simulink model "dyn1"  (R2021b)
settings: Solver=VariableStepAuto  StartTime=0.0  StopTime=10.0  RelTol=1e-3
InitFcn:
  | m=5;
  | I=[0.5 0 0; 0 0.5 0; 0 0 1];
  | c_t=0.02;
  | c_m=0.005;
  | h_i=10;
  | g=9.80665;
  | rho=1;
  | omega_hover=sqrt(m*g/(4*0.5*c_t));
  | dlgtitle= 'Flight Mode Selection';
  | prompt='Select the flight mode:';
  | list={'Hover', 'Underactuation by 10%', 'Overactuation of Only Rear Motor by 10%'};
  | [casee,~]=listdlg('PromptString',prompt,'ListString',list,'ListSize',[240,80],'InitialValue',1,'Name','Mode Selection','OKString','Select','SelectionMode','single');
  | if casee==1
  |     omega1=omega_hover;
  |     omega2=omega_hover;
  |     omega3=omega_hover;
  |     omega4=omega_hover;
  | elseif casee==2
  |     omega1=0.9*omega_hover;
  |     omega2=0.9*omega_hover;
  |     omega3=0.9*omega_hover;
  |     omega4=0.9*omega_hover;
  | elseif casee==3
  |     omega1=omega_hover;
  |     omega2=omega_hover;
  |     omega3=1.1*omega_hover;
  |     omega4=omega_hover;
  | end
undefined symbols (not defined in the file or in its folder): X, Y, Z
libraries: sm_lib x32, nesl_utility x11
(part 2 of 2)

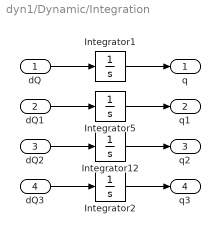
== system dyn1/Dynamic/Integration ==
  dQ : Inport
  dQ1 : Inport  Port=2
  dQ2 : Inport  Port=3
  dQ3 : Inport  Port=4
  Integrator1 : Integrator  InitialCondition=1
  Integrator12 : Integrator
  Integrator2 : Integrator
  Integrator5 : Integrator
  q : Outport
  q1 : Outport  Port=2
  q2 : Outport  Port=3
  q3 : Outport  Port=4
  wires:
  Integrator1/1 -> q/1
  Integrator5/1 -> q1/1
  dQ/1 -> Integrator1/1
  Integrator12/1 -> q2/1
  dQ1/1 -> Integrator5/1
  dQ2/1 -> Integrator12/1
  dQ3/1 -> Integrator2/1
  Integrator2/1 -> q3/1

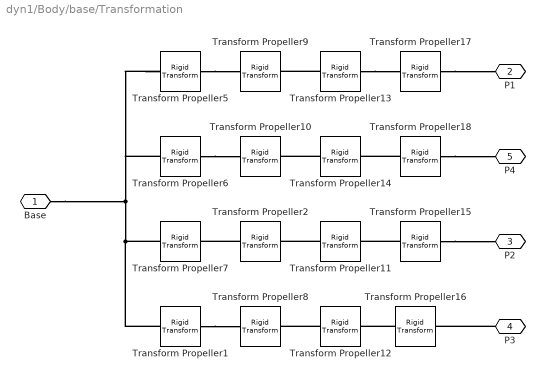
== system dyn1/Body/base/Transformation ==
  Transform Propeller1 : sm_lib/Frames and Transforms/Rigid Transform  TranslationMethod=None  TranslationStandardOffset=45  TranslationLengthUnit=mm  TranslationStandardAxis=+Z  TranslationCartesianOffset=[0 0 -20]  TranslationROffset=0  TranslationROffsetUnits=m  TranslationZOffset=0  TranslationZOffsetUnits=m  TranslationThetaOffset=0  TranslationThetaOffsetUnits=deg  RotationMethod=StandardAxis  RotationAngleUnits=deg  RotationStandardAxis=+Z  RotationAngle=-135  RotationArbitraryAxis=[0 0 1]  FollAlignAxisA=+X  BaseAlignAxisA=+Y  FollAlignAxisB=+Y  BaseAlignAxisB=+Z  RotationSequenceAxes=FollowerAxes  RotationSequence=XYX  RotationSequenceAngles=[0 0 0]  RotationSequenceAnglesUnits=deg  RotationMatrix=[1 0 0; 0 1 0; 0 0 1]
  Transform Propeller{2,8..10} (4 alike) : sm_lib/Frames and Transforms/Rigid Transform  TranslationMethod=StandardAxis  TranslationStandardOffset=60.2  TranslationLengthUnit=mm  TranslationStandardAxis=+X  TranslationCartesianOffset=[0 0 -20]  TranslationROffset=0  TranslationROffsetUnits=m  TranslationZOffset=0  TranslationZOffsetUnits=m  TranslationThetaOffset=0  TranslationThetaOffsetUnits=deg  RotationMethod=None  RotationAngleUnits=deg  RotationStandardAxis=+X  RotationAngle=0  RotationArbitraryAxis=[0 0 1]  FollAlignAxisA=+X  BaseAlignAxisA=+Y  FollAlignAxisB=+Y  BaseAlignAxisB=+Z  RotationSequenceAxes=FollowerAxes  RotationSequence=XYX  RotationSequenceAngles=[0 0 0]  RotationSequenceAnglesUnits=deg  RotationMatrix=[1 0 0; 0 1 0; 0 0 1]
  Transform Propeller{11..14} (4 alike) : sm_lib/Frames and Transforms/Rigid Transform  TranslationMethod=None  TranslationStandardOffset=45  TranslationLengthUnit=mm  TranslationStandardAxis=-Z  TranslationCartesianOffset=[0 0 -20]  TranslationROffset=0  TranslationROffsetUnits=m  TranslationZOffset=0  TranslationZOffsetUnits=m  TranslationThetaOffset=0  TranslationThetaOffsetUnits=deg  RotationMethod=StandardAxis  RotationAngleUnits=deg  RotationStandardAxis=+Y  RotationAngle=180  RotationArbitraryAxis=[0 0 1]  FollAlignAxisA=+X  BaseAlignAxisA=+Y  FollAlignAxisB=+Y  BaseAlignAxisB=+Z  RotationSequenceAxes=FollowerAxes  RotationSequence=XYX  RotationSequenceAngles=[0 0 0]  RotationSequenceAnglesUnits=deg  RotationMatrix=[1 0 0; 0 1 0; 0 0 1]
  Transform Propeller{15..18} (4 alike) : sm_lib/Frames and Transforms/Rigid Transform  TranslationMethod=StandardAxis  TranslationStandardOffset=6  TranslationLengthUnit=mm  TranslationStandardAxis=+Z  TranslationCartesianOffset=[0 0 -20]  TranslationROffset=0  TranslationROffsetUnits=m  TranslationZOffset=0  TranslationZOffsetUnits=m  TranslationThetaOffset=0  TranslationThetaOffsetUnits=deg  RotationMethod=None  RotationAngleUnits=deg  RotationStandardAxis=+X  RotationAngle=0  RotationArbitraryAxis=[0 0 1]  FollAlignAxisA=+X  BaseAlignAxisA=+Y  FollAlignAxisB=+Y  BaseAlignAxisB=+Z  RotationSequenceAxes=FollowerAxes  RotationSequence=XYX  RotationSequenceAngles=[0 0 0]  RotationSequenceAnglesUnits=deg  RotationMatrix=[1 0 0; 0 1 0; 0 0 1]
  Transform Propeller5 : sm_lib/Frames and Transforms/Rigid Transform  TranslationMethod=None  TranslationStandardOffset=135  TranslationLengthUnit=mm  TranslationStandardAxis=+Z  TranslationCartesianOffset=[0 0 -20]  TranslationROffset=0  TranslationROffsetUnits=m  TranslationZOffset=0  TranslationZOffsetUnits=m  TranslationThetaOffset=0  TranslationThetaOffsetUnits=deg  RotationMethod=StandardAxis  RotationAngleUnits=deg  RotationStandardAxis=+Z  RotationAngle=45  RotationArbitraryAxis=[0 0 1]  FollAlignAxisA=+X  BaseAlignAxisA=+Y  FollAlignAxisB=+Y  BaseAlignAxisB=+Z  RotationSequenceAxes=FollowerAxes  RotationSequence=XYX  RotationSequenceAngles=[0 0 0]  RotationSequenceAnglesUnits=deg  RotationMatrix=[1 0 0; 0 1 0; 0 0 1]
  Transform Propeller6 : sm_lib/Frames and Transforms/Rigid Transform  TranslationMethod=None  TranslationStandardOffset=45  TranslationLengthUnit=mm  TranslationStandardAxis=+Z  TranslationCartesianOffset=[0 0 -20]  TranslationROffset=0  TranslationROffsetUnits=m  TranslationZOffset=0  TranslationZOffsetUnits=m  TranslationThetaOffset=0  TranslationThetaOffsetUnits=deg  RotationMethod=StandardAxis  RotationAngleUnits=deg  RotationStandardAxis=+Z  RotationAngle=135  RotationArbitraryAxis=[0 0 1]  FollAlignAxisA=+X  BaseAlignAxisA=+Y  FollAlignAxisB=+Y  BaseAlignAxisB=+Z  RotationSequenceAxes=FollowerAxes  RotationSequence=XYX  RotationSequenceAngles=[0 0 0]  RotationSequenceAnglesUnits=deg  RotationMatrix=[1 0 0; 0 1 0; 0 0 1]
  Transform Propeller7 : sm_lib/Frames and Transforms/Rigid Transform  TranslationMethod=None  TranslationStandardOffset=45  TranslationLengthUnit=mm  TranslationStandardAxis=-Z  TranslationCartesianOffset=[0 0 -20]  TranslationROffset=0  TranslationROffsetUnits=m  TranslationZOffset=0  TranslationZOffsetUnits=m  TranslationThetaOffset=0  TranslationThetaOffsetUnits=deg  RotationMethod=StandardAxis  RotationAngleUnits=deg  RotationStandardAxis=+Z  RotationAngle=-45  RotationArbitraryAxis=[0 0 1]  FollAlignAxisA=+X  BaseAlignAxisA=+Y  FollAlignAxisB=+Y  BaseAlignAxisB=+Z  RotationSequenceAxes=FollowerAxes  RotationSequence=XYX  RotationSequenceAngles=[0 0 0]  RotationSequenceAnglesUnits=deg  RotationMatrix=[1 0 0; 0 1 0; 0 0 1]
  Base : PMIOPort  Side=Left
  P1 : PMIOPort  Port=2  Side=Right
  P2 : PMIOPort  Port=3  Side=Right
  P3 : PMIOPort  Port=4  Side=Right
  P4 : PMIOPort  Port=5  Side=Right
  connections:
  Transform Propeller7/LConn1 -- Base/RConn1 -- Transform Propeller6/LConn1 -- Transform Propeller5/LConn1 -- Transform Propeller1/LConn1
  Transform Propeller2/LConn1 -- Transform Propeller7/RConn1
  Transform Propeller12/LConn1 -- Transform Propeller8/RConn1
  Transform Propeller13/LConn1 -- Transform Propeller9/RConn1
  Transform Propeller11/LConn1 -- Transform Propeller2/RConn1
  Transform Propeller15/LConn1 -- Transform Propeller11/RConn1
  Transform Propeller1/RConn1 -- Transform Propeller8/LConn1
  Transform Propeller14/LConn1 -- Transform Propeller10/RConn1
  Transform Propeller18/RConn1 -- P4/RConn1
  Transform Propeller5/RConn1 -- Transform Propeller9/LConn1
  P3/RConn1 -- Transform Propeller16/RConn1
  Transform Propeller13/RConn1 -- Transform Propeller17/LConn1
  Transform Propeller16/LConn1 -- Transform Propeller12/RConn1
  Transform Propeller18/LConn1 -- Transform Propeller14/RConn1
  Transform Propeller6/RConn1 -- Transform Propeller10/LConn1
  Transform Propeller17/RConn1 -- P1/RConn1
  Transform Propeller15/RConn1 -- P2/RConn1

== matlab function dyn1/Dynamic/MATLAB Function ==
  data: m input; rho input; c_t input; w input; ddx output; ddy output; ddz output; q0 input; q1 input; q2 input; q3 input
function [ddx, ddy, ddz] = forcebalance(m, rho, c_t, w, q0,q1,q2,q3)
w1=w(1)^2;w2=w(2)^2;w3=w(3)^2;w4=w(4)^2;
g=9.80665;
R= [q0^2+q1^2-q2^2-q3^2 2*(q1*q2-q0*q3)      2*(q1*q3+q0*q2);...
         2*(q1*q2+q0*q3)     q0^2-q1^2+q2^2-q3^2  2*(q2*q3-q0*q1);...
         2*(q1*q3-q0*q2)     2*(q2*q3+q0*q1)      q0^2-q1^2-q2^2+q3^2];
F = R*[0;0;-0.5*c_t*rho*(w1+w2+w3+w4)]+m*[0;0;g];
ddx=F(1)/m;
ddy=F(2)/m;
ddz=F(3)/m;

== matlab function dyn1/Dynamic/MATLAB Function1 ==
  data: q input; euler output
function euler  = quat2euler(q)
q0=q(1);q1=q(2);q2=q(3);q3=q(4);
phi = atan2(2*(q0*q1 + q2*q3), 1-2*(q1^2 + q2^2));
theta =-pi/2 + 2*atan2(sqrt(1+2*(q0*q2-q1*q3)),sqrt(1-2*(q0*q2-q1*q3))); %asin(2*(q0*q2 - q3*q1));
si = atan2(2*(q0*q3 + q1*q2), 1-2*(q2^2 + q3^2));
euler=[phi;theta;si];

== matlab function dyn1/Dynamic/MATLAB Function2 ==
  data: p input; q input; r input; I input; w input; rho input; dp output; c_m input; c_t input; dq output; dr output
function  [dp,dq,dr]= momentbalance(p,q,r,I,w,rho,c_m,c_t)
w1=w(1);w2=w(2);w3=w(3);w4=w(4);
S=[0 -r q;r 0 -p;-q p 0];
omwga=[p;q;r];
dd=I\(-S*I*omwga+[.2*(.5*rho*c_t)*(w2-w4);.2*(.5*rho*c_t)*(w1-w3);(.5*rho*c_m)*(w1-w2+w3-w4)]);
dp=dd(1);
dq=dd(2);
dr=dd(3);

== matlab function dyn1/Dynamic/MATLAB Function4 ==
  data: p input; q input; r input; q0 input; q1 input; q2 input; q3 input; dq0 output; dq1 output; dq2 output; dq3 output
function [dq0,dq1,dq2,dq3]=rpy2quat(p,q,r,q0,q1,q2,q3)
B=.5*[0 -p -q -r;p 0 r -q;q -r 0 p;r q -p 0];
angvel=[q0;q1;q2;q3];
a=(B*angvel);
dq0=a(1);
dq1=a(2);
dq2=a(3);
dq3=a(4);
